simulink model "Pulsed_Power_Circuit"  (R2020a)
settings: Solver=VariableStepAuto  StartTime=0.0  StopTime=0.1  RelTol=1e-3
libraries: fl_lib x18, nesl_utility x8, ee_lib x6
settings Model: Creator=mgfee  LastModifiedBy=mgfee
settings SimscapeCC: SimscapeLogType=all

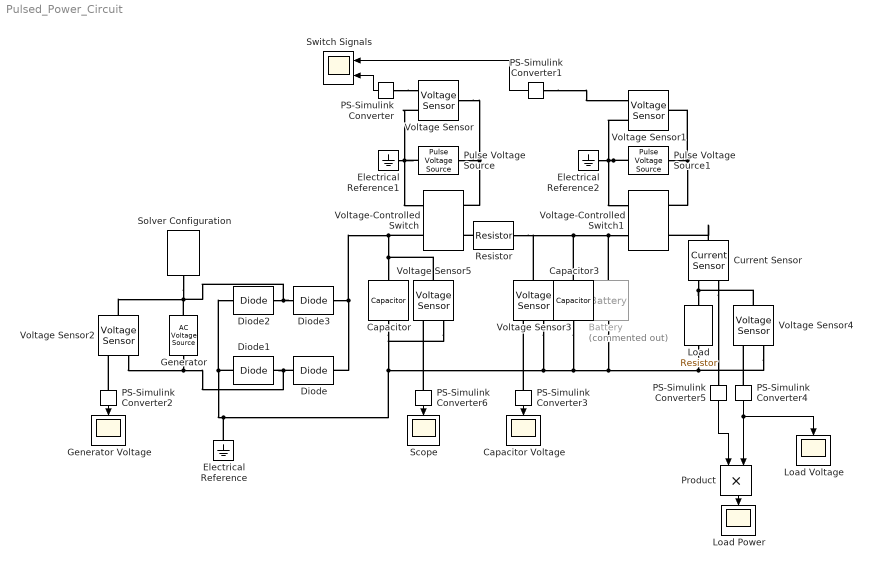
== system Pulsed_Power_Circuit ==
  Battery : ee_lib/Sources/Battery  Commented=on  Vnom=12 V  R1=2 Ohm  prm_AH=1  AH=14083 hr*A  V1=11.5 V  AH1=25 hr*A  prm_R2=2  R2=2000 Ohm  prm_dyn=1  Rp1=0.005 Ohm  tau1=30 s  Rp2=0.005 Ohm  tau2=30 s  Rp3=0.005 Ohm  tau3=30 s  Rp4=0.005 Ohm  tau4=30 s  Rp5=0.005 Ohm  tau5=30 s  prm_fade=1  N_fade=100  AH_fade=45 hr*A  R1_fade=2.02 Ohm  V1_fade=10.35 V  i_specify=off  i_priority=None  i=0 A  i_nominal_specify=off  i_nominal_unit=A  i_nominal_value=1  v_specify=off  v_priority=None  v=0 V  v_nominal_specify=off  v_nominal_unit=V  v_nominal_value=1  charge_specify=off  charge_priority=High  charge=50 hr*A  charge_nominal_specify=off  charge_nominal_unit=hr*A  charge_nominal_value=1  num_cycles_specify=off  num_cycles_priority=High  num_cycles=0  num_cycles_nominal_specify=off  num_cycles_nominal_unit=1  num_cycles_nominal_value=1  thermal_mass=30000 J/K  Tmeas=298.15 K  Vnom_T2=12 V  R1_T2=2.2 Ohm  V1_T2=11.4 V  R2_T2=2200 Ohm  Rp1_T2=0.005 Ohm  tau1_T2=30 s  Rp2_T2=0.005 Ohm  tau2_T2=30 s  Rp3_T2=0.005 Ohm  tau3_T2=30 s  Rp4_T2=0.005 Ohm  tau4_T2=30 s  Rp5_T2=0.005 Ohm  tau5_T2=30 s  Tmeas2=273.15 K  temperature_specify=off  temperature_priority=High  temperature=298.15 K  temperature_nominal_specify=off  temperature_nominal_unit=K  temperature_nominal_value=1
  Capacitor : fl_lib/Electrical/Electrical Elements/Capacitor  c=1e-6 F  r=1e-6 Ohm  g=0 1/Ohm  i_specify=off  i_priority=None  i=0 A  i_nominal_specify=off  i_nominal_unit=A  i_nominal_value=1  v_specify=off  v_priority=None  v=0 V  v_nominal_specify=off  v_nominal_unit=V  v_nominal_value=1  vc_specify=off  vc_priority=High  vc=0 V  vc_nominal_specify=off  vc_nominal_unit=V  vc_nominal_value=1
  Capacitor Voltage : Scope
  Capacitor3 : fl_lib/Electrical/Electrical Elements/Capacitor  c=0.3 F  r=1e-6 Ohm  g=0 1/Ohm  i_specify=off  i_priority=None  i=0 A  i_nominal_specify=off  i_nominal_unit=A  i_nominal_value=1  v_specify=off  v_priority=None  v=0 V  v_nominal_specify=off  v_nominal_unit=V  v_nominal_value=1  vc_specify=off  vc_priority=High  vc=0 V  vc_nominal_specify=off  vc_nominal_unit=V  vc_nominal_value=1
  Current Sensor : fl_lib/Electrical/Electrical Sensors/Current Sensor
  Diode{,1..3} (4 alike) : fl_lib/Electrical/Electrical Elements/Diode  Vf=0.6 V  Ron=0.3 Ohm  Goff=1e-8 1/Ohm  i_specify=off  i_priority=None  i=0 A  i_nominal_specify=off  i_nominal_unit=A  i_nominal_value=1  v_specify=off  v_priority=None  v=0 V  v_nominal_specify=off  v_nominal_unit=V  v_nominal_value=1
  Electrical Reference : fl_lib/Electrical/Electrical Elements/Electrical Reference
  Electrical Reference1 : fl_lib/Electrical/Electrical Elements/Electrical Reference
  Electrical Reference2 : fl_lib/Electrical/Electrical Elements/Electrical Reference
  Generator : fl_lib/Electrical/Electrical Sources/AC Voltage Source  amp=20 V  shift=0 deg  frequency=60 Hz  omega=0 rad/s
  Generator Voltage : Scope
  Load : fl_lib/Electrical/Electrical Elements/Resistor  R=0.1 Ohm  i_specify=off  i_priority=None  i=0 A  i_nominal_specify=off  i_nominal_unit=A  i_nominal_value=1  v_specify=off  v_priority=None  v=0 V  v_nominal_specify=off  v_nominal_unit=V  v_nominal_value=1
  Load Power : Scope
  Load Voltage : Scope
  PS-Simulink Converter{,1..6} (7 alike) : nesl_utility/PS-Simulink Converter  PhysicalDomain=network_engine_domain  SubClassName=ps_output  LeftPortType=input  RightPortType=output  PseudoPeriodic=off  Frequencies=[]  Unit=inherit  AffineConversion=off
  Product : Product
  Pulse Voltage Source : ee_lib/Additional Components/SPICE Sources/Pulse Voltage Source  V1=0 V  V2=1 V  TD=0 s  TR=1e-9 s  TF=1e-9 s  PW=5 ms  PER=10 ms
      settings: SourceProductBaseCode=PS  InternalSimscapePortConfiguration="{\"Bottom\":[],\"Left\":[{\"id\":\"p\",\"label\":\"\",\"type\":\"foundation.electrical.electrical\"}],\"Right\":[{\"id\":\"n\",\"label\":\"\",\"type\":\"foundation.electrical.electrical\"}],\"Top\":[]}"
  Pulse Voltage Source1 : ee_lib/Additional Components/SPICE Sources/Pulse Voltage Source  V1=0 V  V2=1 V  TD=5 ms  TR=1e-9 s  TF=1e-9 s  PW=1 ms  PER=10 ms
      settings: SourceProductBaseCode=PS  InternalSimscapePortConfiguration="{\"Bottom\":[],\"Left\":[{\"id\":\"p\",\"label\":\"\",\"type\":\"foundation.electrical.electrical\"}],\"Right\":[{\"id\":\"n\",\"label\":\"\",\"type\":\"foundation.electrical.electrical\"}],\"Top\":[]}"
  Resistor : ee_lib/Passive/Resistor  R=1e-6 Ohm  R_tol=5  enable_R_tol=0  tol_distribution=1  nSigma=4  enable_operating_limits=0  operating_limit_action=2  max_working_voltage=100 V  power_rating=1 W  enable_faults=0  fault_action=1  R_faulted=inf Ohm  enable_temporal_fault=0  t_fault=1 s  enable_behavioral_fault=0  max_permissible_current=1 A  t_fail_on_current=1 s  noise_mode=0  sample_time=1e-3 s  repeatability=1  auto_seed=1105989530  user_seed=0  Tdevice=25 degC  alpha=3.93e-3 1/K  Tmeas=25 degC  thermal_mass=100 J/K  power_derating_T1=70 degC  power_derating_T2=155 degC  operating_temperature_range_vec=[-50, 150] degC  temperature_specify=off  temperature_priority=High  temperature=298.15 K  temperature_nominal_specify=off  temperature_nominal_unit=K  temperature_nominal_value=1
  Scope : Scope
  Solver Configuration : nesl_utility/Solver Configuration  PhysicalDomain=network_engine_domain  SubClassName=solver  LeftPortType=input  RightPortType=generic  Tones=[]  Harmonics=[]  SimulateNoise=off  Profile=off  UseLocalSampling=off  EnableSwitchedLinearOptims=on  FrequencyDomain=off  UseCCode=off  RelTol=0.001  AbsTol=1e-06  MinStep=1e-09  ToWorkspace=off  RevertToSquareIcSolve=off  NumHomotopyIterations=100  PhasorMode=off  PhasorModeNumHarmonics=1  DoDC=off  ResidualTolerance=1e-09  UseLocalSolver=off  LocalSolverChoice=NE_BACKWARD_EULER_ADVANCER  LocalSolverSampleTime=0.001  DoFixedCost=off  MaxNonlinIter=3  MaxModeIter=2  LinearAlgebra=auto  EquationFormulation=NE_TIME_EF  DelaysMemoryBudget=1024  AutomaticFiltering=on  FilteringTimeConstant=0.001  PartitionStorageMethod=AS_NEEDED  PartitionMemoryBudget=1024  PartitionMethod=ROBUST
  Switch Signals : Scope  NumInputPorts=2
  Voltage Sensor{,1..5} (6 alike) : fl_lib/Electrical/Electrical Sensors/Voltage Sensor
  Voltage-Controlled Switch : ee_lib/Additional Components/SPICE Passives/Voltage-Controlled Switch  VT=0.5 V  VH=0 V  RON=1 Ohm  ROFF=1e12 Ohm  IC_state=1
      settings: SourceProductBaseCode=PS  InternalSimscapePortConfiguration="{\"Bottom\":[],\"Left\":[{\"id\":\"p1\",\"label\":\"1+\",\"type\":\"foundation.electrical.electrical\"},{\"id\":\"p2\",\"label\":\"2+\",\"type\":\"foundation.electrical.electrical\"}],\"Right\":[{\"id\":\"n1\",\"label\":\"1-\",\"type\":\"foundation.electrical.electrical\"},{\"id\":\"n2\",\"label\":\"2-\",\"type\":\"foundation.electrical.electrical\"}],\"Top\":[]}"
  Voltage-Controlled Switch1 : ee_lib/Additional Components/SPICE Passives/Voltage-Controlled Switch  VT=.5 V  VH=0 V  RON=1 Ohm  ROFF=1e12 Ohm  IC_state=1
      settings: SourceProductBaseCode=PS  InternalSimscapePortConfiguration="{\"Bottom\":[],\"Left\":[{\"id\":\"p1\",\"label\":\"1+\",\"type\":\"foundation.electrical.electrical\"},{\"id\":\"p2\",\"label\":\"2+\",\"type\":\"foundation.electrical.electrical\"}],\"Right\":[{\"id\":\"n1\",\"label\":\"1-\",\"type\":\"foundation.electrical.electrical\"},{\"id\":\"n2\",\"label\":\"2-\",\"type\":\"foundation.electrical.electrical\"}],\"Top\":[]}"
  wires:
  PS-Simulink Converter1/1 -> Switch Signals/1
  PS-Simulink Converter/1 -> Switch Signals/2
  PS-Simulink Converter2/1 -> Generator Voltage/1
  PS-Simulink Converter3/1 -> Capacitor Voltage/1
  PS-Simulink Converter4/1 -> Product/2, Load Voltage/1
  PS-Simulink Converter5/1 -> Product/1
  Product/1 -> Load Power/1
  PS-Simulink Converter6/1 -> Scope/1
  connections:
  Diode2/RConn1 -- Solver Configuration/RConn1 -- Generator/LConn1 -- Voltage Sensor2/LConn1 -- Diode3/LConn1
  Diode1/LConn1 -- Diode2/LConn1 -- Electrical Reference/LConn1 -- Voltage Sensor5/RConn2 -- Capacitor/RConn1 -- Voltage Sensor3/RConn2 -- Capacitor3/RConn1 -- Voltage Sensor4/RConn2 -- Load/RConn1 -- Battery/RConn1
  Capacitor3/LConn1 -- Voltage Sensor3/LConn1 -- Resistor/RConn1 -- Voltage-Controlled Switch1/RConn2 -- Battery/LConn1
  Voltage Sensor4/LConn1 -- Current Sensor/RConn2 -- Load/LConn1
  Pulse Voltage Source/LConn1 -- Voltage Sensor/LConn1 -- Voltage-Controlled Switch/LConn1
  Pulse Voltage Source1/LConn1 -- Voltage Sensor1/LConn1 -- Voltage-Controlled Switch1/LConn1
  Pulse Voltage Source1/RConn1 -- Voltage-Controlled Switch1/RConn1 -- Voltage Sensor1/RConn2 -- Electrical Reference2/LConn1
  Pulse Voltage Source/RConn1 -- Electrical Reference1/LConn1 -- Voltage Sensor/RConn2 -- Voltage-Controlled Switch/RConn1
  PS-Simulink Converter/LConn1 -- Voltage Sensor/RConn1
  PS-Simulink Converter1/LConn1 -- Voltage Sensor1/RConn1
  PS-Simulink Converter2/LConn1 -- Voltage Sensor2/RConn1
  PS-Simulink Converter3/LConn1 -- Voltage Sensor3/RConn1
  PS-Simulink Converter4/LConn1 -- Voltage Sensor4/RConn1
  Current Sensor/LConn1 -- Voltage-Controlled Switch1/LConn2
  Current Sensor/RConn1 -- PS-Simulink Converter5/LConn1
  Diode3/RConn1 -- Diode/RConn1 -- Voltage-Controlled Switch/RConn2 -- Voltage Sensor5/LConn1 -- Capacitor/LConn1
  PS-Simulink Converter6/LConn1 -- Voltage Sensor5/RConn1
  Resistor/LConn1 -- Voltage-Controlled Switch/LConn2
  Voltage Sensor2/RConn2 -- Generator/RConn1 -- Diode/LConn1 -- Diode1/RConn1
